simulink model "RoboBoat_SS_July3_v6"  (R2014a)
settings: Solver=FixedStepDiscrete  StartTime=0.0  StopTime=inf  FixedStep=.1  RelTol=1e-3
undefined symbols (not defined in the file): Com1, Com2, Com3, Com4, DiscIntNeverNeededParam, standard
libraries: xpcseriallib x29, visiontextngfix x25, simulink x20, slrtlib x7, speedgoatlib_IO102 x5, speedgoatlib x1
(part 3 of 5)

== system RoboBoat_SS_July3_v6/Main FSM/Obstacle Navigation1/Enter Gate/Gate 2 (White & White) ==
  Sensors : Inport
  RGB image : Inport  Port=2
  Enable : EnablePort  ShowOutputPort=on
  Bus Selector : BusSelector  OutputSignals=Serial In.Buoy Info.Probability,Serial In.Buoy Info.Color ID,Serial In.Buoy Info.Distance,Serial In.Buoy Info.Angle,Serial In.Compass.Heading,Serial In.GPS.latitude,Serial In.GPS.longitude
  Compare To Constant : simulink/Logic and Bit Operations/Compare To Constant  relop=<=  const=2  OutDataTypeStr=boolean
  Compare To Constant1 : simulink/Logic and Bit Operations/Compare To Constant  relop=>=  const=120  OutDataTypeStr=boolean
  Data Type Conversion2 : DataTypeConversion  OutDataTypeStr=double
  Discrete-Time Integrator : DiscreteIntegrator  SampleTime=.1  ICPrevOutput=DiscIntNeverNeededParam  ICPrevScaledInput=DiscIntNeverNeededParam
  Distance : MATLAB Function  TreatAsAtomicUnit=on
  Insert Text : visiontextngfix/Insert Text  inputType=Obsolete  theText='Enter Gate 2'  getTextLocFrom=Specify via dialog  textLoc=[1 1]  getTextColorFrom=Specify via dialog  textColor=[0 0 0]  getTextIntensityFrom=Specify via dialog  textIntensity=0  getTextOpacityFrom=Specify via dialog  textOpacity=1.0  dummyVar2=0  dummyVar3=0  dummyVar4=0  imagePorts=One multidimensional signal  isInputTransposed=off  fontFace=LucidaSansRegular  dummyVar1=0  blockFontSize=12  antiAliased=on
  Logical Operator : Logic  Operator=OR  AllPortsSameDT=off  OutDataTypeStr=boolean
  MATLAB Function : MATLAB Function  TreatAsAtomicUnit=on
  Output Heirarchy : Subsystem
  Outputs : Outport
  wires:
  Output Heirarchy/1(Outputs) -> Outputs/1
  Sensors/1 -> Output Heirarchy/2(Sensors), Bus Selector/1
  Bus Selector/1 -> MATLAB Function/1(Prob)  "<Probability>"
  Bus Selector/2 -> MATLAB Function/2(ColorID)  "<Color ID>"
  Bus Selector/3 -> MATLAB Function/3(Dist)  "<Distance>"
  Bus Selector/4 -> MATLAB Function/4(Ang)  "<Angle>"
  Bus Selector/5 -> MATLAB Function/5(CurrentHeading)  "<Heading>"
  Enable/1 -> Discrete-Time Integrator/1
  Discrete-Time Integrator/1 -> Compare To Constant1/1, MATLAB Function/8(Timer)
  MATLAB Function/1(RPM) -> Output Heirarchy/3(RPM)
  MATLAB Function/2(DesiredHeading) -> Output Heirarchy/4(Desired Heading)
  Bus Selector/6 -> MATLAB Function/6(GPSLat), Distance/2(GPSLat)  "<latitude>"
  Bus Selector/7 -> MATLAB Function/7(GPSLong), Distance/3(GPSLong)  "<longitude>"
  Distance/1(Distance) -> Compare To Constant/1
  RGB image/1 -> Insert Text/1
  Data Type Conversion2/1 -> Output Heirarchy/5(Task Finished)
  Compare To Constant/1 -> Logical Operator/2
  MATLAB Function/3(gateGPS) -> Distance/1(DesiredGPS)
  Compare To Constant1/1 -> Logical Operator/1
  Logical Operator/1 -> Data Type Conversion2/1
  Insert Text/1 -> Output Heirarchy/1(Annotated Image)

== system RoboBoat_SS_July3_v6/Main FSM/Obstacle Navigation1/Enter Gate/Gate 3 (White & Green) ==
  Sensors : Inport
  RGB image : Inport  Port=2
  Enable : EnablePort  ShowOutputPort=on
  Bus Selector : BusSelector  OutputSignals=Serial In.Buoy Info.Probability,Serial In.Buoy Info.Color ID,Serial In.Buoy Info.Distance,Serial In.Buoy Info.Angle,Serial In.Compass.Heading,Serial In.GPS.latitude,Serial In.GPS.longitude
  Compare To Constant : simulink/Logic and Bit Operations/Compare To Constant  relop=<=  const=2  OutDataTypeStr=boolean
  Compare To Constant1 : simulink/Logic and Bit Operations/Compare To Constant  relop=>=  const=120  OutDataTypeStr=boolean
  Data Type Conversion2 : DataTypeConversion  OutDataTypeStr=double
  Discrete-Time Integrator : DiscreteIntegrator  SampleTime=.1  ICPrevOutput=DiscIntNeverNeededParam  ICPrevScaledInput=DiscIntNeverNeededParam
  Distance : MATLAB Function  TreatAsAtomicUnit=on
  Insert Text : visiontextngfix/Insert Text  inputType=Obsolete  theText='Enter Gate 3'  getTextLocFrom=Specify via dialog  textLoc=[1 1]  getTextColorFrom=Specify via dialog  textColor=[0 0 0]  getTextIntensityFrom=Specify via dialog  textIntensity=0  getTextOpacityFrom=Specify via dialog  textOpacity=1.0  dummyVar2=0  dummyVar3=0  dummyVar4=0  imagePorts=One multidimensional signal  isInputTransposed=off  fontFace=LucidaSansRegular  dummyVar1=0  blockFontSize=12  antiAliased=on
  Logical Operator : Logic  Operator=OR  AllPortsSameDT=off  OutDataTypeStr=boolean
  MATLAB Function : MATLAB Function  TreatAsAtomicUnit=on
  Output Heirarchy : Subsystem
  Outputs : Outport
  wires:
  Output Heirarchy/1(Outputs) -> Outputs/1
  Sensors/1 -> Output Heirarchy/2(Sensors), Bus Selector/1
  Bus Selector/1 -> MATLAB Function/1(Prob)  "<Probability>"
  Bus Selector/2 -> MATLAB Function/2(ColorID)  "<Color ID>"
  Bus Selector/3 -> MATLAB Function/3(Dist)  "<Distance>"
  Bus Selector/4 -> MATLAB Function/4(Ang)  "<Angle>"
  Bus Selector/5 -> MATLAB Function/5(CurrentHeading)  "<Heading>"
  Enable/1 -> Discrete-Time Integrator/1
  Discrete-Time Integrator/1 -> Compare To Constant1/1, MATLAB Function/8(Timer)
  MATLAB Function/1(RPM) -> Output Heirarchy/3(RPM)
  MATLAB Function/2(DesiredHeading) -> Output Heirarchy/4(Desired Heading)
  Bus Selector/6 -> MATLAB Function/6(GPSLat), Distance/2(GPSLat)  "<latitude>"
  Bus Selector/7 -> MATLAB Function/7(GPSLong), Distance/3(GPSLong)  "<longitude>"
  Distance/1(Distance) -> Compare To Constant/1
  RGB image/1 -> Insert Text/1
  Data Type Conversion2/1 -> Output Heirarchy/5(Task Finished)
  Compare To Constant/1 -> Logical Operator/2
  MATLAB Function/3(gateGPS) -> Distance/1(DesiredGPS)
  Compare To Constant1/1 -> Logical Operator/1
  Logical Operator/1 -> Data Type Conversion2/1
  Insert Text/1 -> Output Heirarchy/1(Annotated Image)

== system RoboBoat_SS_July3_v6/Main FSM/Obstacle Navigation1/Enter Gate/Output Reassign ==
  Outputs in : Inport
  Bus Assignment : BusAssignment  AssignedSignals=Task Finished
  Bus Selector : BusSelector  OutputSignals=Task Finished
  Constant : Constant  Value=0
  Outputs : Outport
  Finished : Outport  Port=2
  wires:
  Outputs in/1 -> Bus Assignment/1, Bus Selector/1
  Bus Selector/1 -> Finished/1  "<Task Finished>"
  Bus Assignment/1 -> Outputs/1
  Constant/1 -> Bus Assignment/2

== system RoboBoat_SS_July3_v6/Main FSM/Obstacle Navigation1/Exit Gate/Gate 1 (Red & White) ==
  Sensors : Inport
  RGB image : Inport  Port=2
  Enable : EnablePort  ShowOutputPort=on
  Bus Selector : BusSelector  OutputSignals=Serial In.Buoy Info.Probability,Serial In.Buoy Info.Color ID,Serial In.Buoy Info.Distance,Serial In.Buoy Info.Angle,Serial In.Compass.Heading,Serial In.GPS.latitude,Serial In.GPS.longitude
  Compare To Constant : simulink/Logic and Bit Operations/Compare To Constant  relop=<=  const=2  OutDataTypeStr=boolean
  Compare To Constant1 : simulink/Logic and Bit Operations/Compare To Constant  relop=>=  const=120  OutDataTypeStr=boolean
  Data Type Conversion2 : DataTypeConversion  OutDataTypeStr=double
  Discrete-Time Integrator : DiscreteIntegrator  SampleTime=.1  ICPrevOutput=DiscIntNeverNeededParam  ICPrevScaledInput=DiscIntNeverNeededParam
  Distance : MATLAB Function  TreatAsAtomicUnit=on
  Insert Text : visiontextngfix/Insert Text  inputType=Obsolete  theText='Exit Gate 1'  getTextLocFrom=Specify via dialog  textLoc=[1 1]  getTextColorFrom=Specify via dialog  textColor=[0 0 0]  getTextIntensityFrom=Specify via dialog  textIntensity=0  getTextOpacityFrom=Specify via dialog  textOpacity=1.0  dummyVar2=0  dummyVar3=0  dummyVar4=0  imagePorts=One multidimensional signal  isInputTransposed=off  fontFace=LucidaSansRegular  dummyVar1=0  blockFontSize=12  antiAliased=on
  Logical Operator : Logic  Operator=OR  AllPortsSameDT=off  OutDataTypeStr=boolean
  MATLAB Function : MATLAB Function  TreatAsAtomicUnit=on
  Output Heirarchy : Subsystem
  Outputs : Outport
  wires:
  Output Heirarchy/1(Outputs) -> Outputs/1
  Sensors/1 -> Output Heirarchy/2(Sensors), Bus Selector/1
  Bus Selector/1 -> MATLAB Function/1(Prob)  "<Probability>"
  Bus Selector/2 -> MATLAB Function/2(ColorID)  "<Color ID>"
  Bus Selector/3 -> MATLAB Function/3(Dist)  "<Distance>"
  Bus Selector/4 -> MATLAB Function/4(Ang)  "<Angle>"
  Bus Selector/5 -> MATLAB Function/5(CurrentHeading)  "<Heading>"
  Enable/1 -> Discrete-Time Integrator/1
  Discrete-Time Integrator/1 -> Compare To Constant1/1, MATLAB Function/8(Timer)
  MATLAB Function/1(RPM) -> Output Heirarchy/3(RPM)
  MATLAB Function/2(DesiredHeading) -> Output Heirarchy/4(Desired Heading)
  Bus Selector/6 -> MATLAB Function/6(GPSLat), Distance/2(GPSLat)  "<latitude>"
  Bus Selector/7 -> MATLAB Function/7(GPSLong), Distance/3(GPSLong)  "<longitude>"
  Distance/1(Distance) -> Compare To Constant/1
  RGB image/1 -> Insert Text/1
  Insert Text/1 -> Output Heirarchy/1(Annotated Image)
  Data Type Conversion2/1 -> Output Heirarchy/5(Task Finished)
  Compare To Constant/1 -> Logical Operator/2
  MATLAB Function/3(gateGPS) -> Distance/1(DesiredGPS)
  Compare To Constant1/1 -> Logical Operator/1
  Logical Operator/1 -> Data Type Conversion2/1

== system RoboBoat_SS_July3_v6/Main FSM/Obstacle Navigation1/Exit Gate/Gate 2 (White & White) ==
  Sensors : Inport
  RGB image : Inport  Port=2
  Enable : EnablePort  ShowOutputPort=on
  Bus Selector : BusSelector  OutputSignals=Serial In.Buoy Info.Probability,Serial In.Buoy Info.Color ID,Serial In.Buoy Info.Distance,Serial In.Buoy Info.Angle,Serial In.Compass.Heading,Serial In.GPS.latitude,Serial In.GPS.longitude
  Compare To Constant : simulink/Logic and Bit Operations/Compare To Constant  relop=<=  const=2  OutDataTypeStr=boolean
  Compare To Constant1 : simulink/Logic and Bit Operations/Compare To Constant  relop=>=  const=120  OutDataTypeStr=boolean
  Data Type Conversion2 : DataTypeConversion  OutDataTypeStr=double
  Discrete-Time Integrator : DiscreteIntegrator  SampleTime=.1  ICPrevOutput=DiscIntNeverNeededParam  ICPrevScaledInput=DiscIntNeverNeededParam
  Distance : MATLAB Function  TreatAsAtomicUnit=on
  Insert Text : visiontextngfix/Insert Text  inputType=Obsolete  theText='Exit Gate 2'  getTextLocFrom=Specify via dialog  textLoc=[1 1]  getTextColorFrom=Specify via dialog  textColor=[0 0 0]  getTextIntensityFrom=Specify via dialog  textIntensity=0  getTextOpacityFrom=Specify via dialog  textOpacity=1.0  dummyVar2=0  dummyVar3=0  dummyVar4=0  imagePorts=One multidimensional signal  isInputTransposed=off  fontFace=LucidaSansRegular  dummyVar1=0  blockFontSize=12  antiAliased=on
  Logical Operator : Logic  Operator=OR  AllPortsSameDT=off  OutDataTypeStr=boolean
  MATLAB Function : MATLAB Function  TreatAsAtomicUnit=on
  Output Heirarchy : Subsystem
  Outputs : Outport
  wires:
  Output Heirarchy/1(Outputs) -> Outputs/1
  Sensors/1 -> Output Heirarchy/2(Sensors), Bus Selector/1
  Bus Selector/1 -> MATLAB Function/1(Prob)  "<Probability>"
  Bus Selector/2 -> MATLAB Function/2(ColorID)  "<Color ID>"
  Bus Selector/3 -> MATLAB Function/3(Dist)  "<Distance>"
  Bus Selector/4 -> MATLAB Function/4(Ang)  "<Angle>"
  Bus Selector/5 -> MATLAB Function/5(CurrentHeading)  "<Heading>"
  Enable/1 -> Discrete-Time Integrator/1
  Discrete-Time Integrator/1 -> Compare To Constant1/1, MATLAB Function/8(Timer)
  MATLAB Function/1(RPM) -> Output Heirarchy/3(RPM)
  MATLAB Function/2(DesiredHeading) -> Output Heirarchy/4(Desired Heading)
  Bus Selector/6 -> MATLAB Function/6(GPSLat), Distance/2(GPSLat)  "<latitude>"
  Bus Selector/7 -> MATLAB Function/7(GPSLong), Distance/3(GPSLong)  "<longitude>"
  Distance/1(Distance) -> Compare To Constant/1
  RGB image/1 -> Insert Text/1
  Data Type Conversion2/1 -> Output Heirarchy/5(Task Finished)
  Compare To Constant/1 -> Logical Operator/2
  MATLAB Function/3(gateGPS) -> Distance/1(DesiredGPS)
  Compare To Constant1/1 -> Logical Operator/1
  Logical Operator/1 -> Data Type Conversion2/1
  Insert Text/1 -> Output Heirarchy/1(Annotated Image)

== system RoboBoat_SS_July3_v6/Main FSM/Obstacle Navigation1/Exit Gate/Gate 3 (White & Green) ==
  Sensors : Inport
  RGB image : Inport  Port=2
  Enable : EnablePort  ShowOutputPort=on
  Bus Selector : BusSelector  OutputSignals=Serial In.Buoy Info.Probability,Serial In.Buoy Info.Color ID,Serial In.Buoy Info.Distance,Serial In.Buoy Info.Angle,Serial In.Compass.Heading,Serial In.GPS.latitude,Serial In.GPS.longitude
  Compare To Constant : simulink/Logic and Bit Operations/Compare To Constant  relop=<=  const=2  OutDataTypeStr=boolean
  Compare To Constant1 : simulink/Logic and Bit Operations/Compare To Constant  relop=>=  const=120  OutDataTypeStr=boolean
  Data Type Conversion2 : DataTypeConversion  OutDataTypeStr=double
  Discrete-Time Integrator : DiscreteIntegrator  SampleTime=.1  ICPrevOutput=DiscIntNeverNeededParam  ICPrevScaledInput=DiscIntNeverNeededParam
  Distance : MATLAB Function  TreatAsAtomicUnit=on
  Insert Text : visiontextngfix/Insert Text  inputType=Obsolete  theText='Exit Gate 3'  getTextLocFrom=Specify via dialog  textLoc=[1 1]  getTextColorFrom=Specify via dialog  textColor=[0 0 0]  getTextIntensityFrom=Specify via dialog  textIntensity=0  getTextOpacityFrom=Specify via dialog  textOpacity=1.0  dummyVar2=0  dummyVar3=0  dummyVar4=0  imagePorts=One multidimensional signal  isInputTransposed=off  fontFace=LucidaSansRegular  dummyVar1=0  blockFontSize=12  antiAliased=on
  Logical Operator : Logic  Operator=OR  AllPortsSameDT=off  OutDataTypeStr=boolean
  MATLAB Function : MATLAB Function  TreatAsAtomicUnit=on
  Output Heirarchy : Subsystem
  Outputs : Outport
  wires:
  Output Heirarchy/1(Outputs) -> Outputs/1
  Sensors/1 -> Output Heirarchy/2(Sensors), Bus Selector/1
  Bus Selector/1 -> MATLAB Function/1(Prob)  "<Probability>"
  Bus Selector/2 -> MATLAB Function/2(ColorID)  "<Color ID>"
  Bus Selector/3 -> MATLAB Function/3(Dist)  "<Distance>"
  Bus Selector/4 -> MATLAB Function/4(Ang)  "<Angle>"
  Bus Selector/5 -> MATLAB Function/5(CurrentHeading)  "<Heading>"
  Enable/1 -> Discrete-Time Integrator/1
  Discrete-Time Integrator/1 -> Compare To Constant1/1, MATLAB Function/8(Timer)
  MATLAB Function/1(RPM) -> Output Heirarchy/3(RPM)
  MATLAB Function/2(DesiredHeading) -> Output Heirarchy/4(Desired Heading)
  Bus Selector/6 -> MATLAB Function/6(GPSLat), Distance/2(GPSLat)  "<latitude>"
  Bus Selector/7 -> MATLAB Function/7(GPSLong), Distance/3(GPSLong)  "<longitude>"
  Distance/1(Distance) -> Compare To Constant/1
  RGB image/1 -> Insert Text/1
  Data Type Conversion2/1 -> Output Heirarchy/5(Task Finished)
  Compare To Constant/1 -> Logical Operator/2
  MATLAB Function/3(gateGPS) -> Distance/1(DesiredGPS)
  Compare To Constant1/1 -> Logical Operator/1
  Logical Operator/1 -> Data Type Conversion2/1
  Insert Text/1 -> Output Heirarchy/1(Annotated Image)

== system RoboBoat_SS_July3_v6/Main FSM/Obstacle Navigation1/GPS: Center/Approach ==
  Sensors : Inport
  RGB image : Inport  Port=2
  Enable : EnablePort
  Annotate Task : visiontextngfix/Insert Text  inputType=Obsolete  theText='GPS - Center: Approach - Distance: %f'  getTextLocFrom=Specify via dialog  textLoc=[10 70]  getTextColorFrom=Specify via dialog  textColor=[255 0 0]  getTextIntensityFrom=Specify via dialog  textIntensity=0  getTextOpacityFrom=Specify via dialog  textOpacity=1.0  dummyVar2=0  dummyVar3=0  dummyVar4=0  imagePorts=One multidimensional signal  isInputTransposed=off  fontFace=LucidaSansRegular  dummyVar1=0  blockFontSize=12  antiAliased=on
  Annotate Task2 : visiontextngfix/Insert Text  inputType=Obsolete  theText='Obst Nav Start'  getTextLocFrom=Specify via dialog  textLoc=[1 1]  getTextColorFrom=Specify via dialog  textColor=[0 0 0]  getTextIntensityFrom=Specify via dialog  textIntensity=0  getTextOpacityFrom=Specify via dialog  textOpacity=1.0  dummyVar2=0  dummyVar3=0  dummyVar4=0  imagePorts=One multidimensional signal  isInputTransposed=off  fontFace=LucidaSansRegular  dummyVar1=0  blockFontSize=12  antiAliased=on
  Bus Selector : BusSelector  OutputSignals=Serial In.GPS.latitude,Serial In.GPS.longitude
  Compare To Constant : simulink/Logic and Bit Operations/Compare To Constant  relop=<=  const=5  OutDataTypeStr=boolean
  Data Store Read : DataStoreRead  DataStoreName=obstNavStartGPS  SampleTime=0.1
  Data Type Conversion : DataTypeConversion  OutDataTypeStr=double
  Desired Heading and Distance : MATLAB Function  TreatAsAtomicUnit=on
  MATLAB Function : MATLAB Function  Commented=on  TreatAsAtomicUnit=on
  Output Heirarchy : Subsystem
  "Scope " : slrtlib/Displays and Logging/Scope   Commented=on  scopeno=1  scopetype=File  autostart=on  viewmode=Graphical redraw  formatstr='%15.6f'  grid=on  ylimits=[0,0]  nosamples=1200  noprepostsamples=0  interleave=1  triggermode=FreeRun  triggersignal=1  trigsignalfromport=off  triggerlevel=1  triggerslope=Either  triggerscope=1  triggersample=0  filename=ApprLog.dat  mode=Lazy  writesize=512  autorestart=off  dynamicfilemode=off  maxwritefilesize=512*1024^2
  Outputs : Outport
  wires:
  Sensors/1 -> Output Heirarchy/4(Sensors), Bus Selector/1  "Sensors"
  Data Store Read/1 -> Desired Heading and Distance/1(DesiredGPS)
  Bus Selector/1 -> Desired Heading and Distance/2(GPSLat)  "<latitude>"
  Bus Selector/2 -> Desired Heading and Distance/3(GPSLong)  "<longitude>"
  Desired Heading and Distance/2(DesiredHeading) -> Output Heirarchy/2(Desired Heading)
  Annotate Task/1 -> Output Heirarchy/3(Annotated Image)
  RGB image/1 -> Annotate Task2/1
  Output Heirarchy/1(Outputs) -> Outputs/1
  Annotate Task2/1 -> Annotate Task/1
  MATLAB Function/1(out) -> "Scope "/1
  Desired Heading and Distance/1(Distance) -> Compare To Constant/1, Annotate Task/2
  Data Type Conversion/1 -> Output Heirarchy/1(Finished)  "Task Finished"
  Compare To Constant/1 -> Data Type Conversion/1

== system RoboBoat_SS_July3_v6/Main FSM/Obstacle Navigation1/GPS: Center/Orient ==
  Sensors : Inport
  RGB image : Inport  Port=2
  Enable : EnablePort
  Annotate Task : visiontextngfix/Insert Text  inputType=Obsolete  theText='GPS - Center: Orient %f'  getTextLocFrom=Specify via dialog  textLoc=[10 70]  getTextColorFrom=Specify via dialog  textColor=[255 0 0]  getTextIntensityFrom=Specify via dialog  textIntensity=0  getTextOpacityFrom=Specify via dialog  textOpacity=1.0  dummyVar2=0  dummyVar3=0  dummyVar4=0  imagePorts=One multidimensional signal  isInputTransposed=off  fontFace=LucidaSansRegular  dummyVar1=0  blockFontSize=12  antiAliased=on
  Annotate Task1 : visiontextngfix/Insert Text  inputType=Obsolete  theText='Current Heading %f'  getTextLocFrom=Specify via dialog  textLoc=[10 40]  getTextColorFrom=Specify via dialog  textColor=[255 0 0]  getTextIntensityFrom=Specify via dialog  textIntensity=0  getTextOpacityFrom=Specify via dialog  textOpacity=1.0  dummyVar2=0  dummyVar3=0  dummyVar4=0  imagePorts=One multidimensional signal  isInputTransposed=off  fontFace=LucidaSansRegular  dummyVar1=0  blockFontSize=12  antiAliased=on
  Annotate Task2 : visiontextngfix/Insert Text  inputType=Obsolete  theText='Obst Nav Start'  getTextLocFrom=Specify via dialog  textLoc=[1 1]  getTextColorFrom=Specify via dialog  textColor=[0 0 0]  getTextIntensityFrom=Specify via dialog  textIntensity=0  getTextOpacityFrom=Specify via dialog  textOpacity=1.0  dummyVar2=0  dummyVar3=0  dummyVar4=0  imagePorts=One multidimensional signal  isInputTransposed=off  fontFace=LucidaSansRegular  dummyVar1=0  blockFontSize=12  antiAliased=on
  Bus Selector : BusSelector  OutputSignals=Serial In.GPS.latitude,Serial In.GPS.longitude,Serial In.Compass.Heading
  Data Store Read : DataStoreRead  DataStoreName=obstNavStartGPS  SampleTime=0.1
  Desired Heading : MATLAB Function  TreatAsAtomicUnit=on
  Output Heirarchy1 : Subsystem
  Within Range : MATLAB Function  TreatAsAtomicUnit=on
  Outputs : Outport
  Finished : Outport  Port=2
  wires:
  Sensors/1 -> Output Heirarchy1/3(Sensors), Bus Selector/1  "Sensors"
  Data Store Read/1 -> Desired Heading/1(DesiredGPS)
  Bus Selector/1 -> Desired Heading/2(GPSLat)  "<latitude>"
  Bus Selector/2 -> Desired Heading/3(GPSLong)  "<longitude>"
  Desired Heading/1(DesiredHeading) -> Output Heirarchy1/2(Desired Heading), Annotate Task/2, Within Range/1(DesiredHeading)
  Bus Selector/3 -> Annotate Task1/2, Within Range/2(Compass)  "<Heading>"
  Within Range/1(Finished) -> Finished/1
  RGB image/1 -> Annotate Task2/1
  Output Heirarchy1/1(Outputs) -> Outputs/1
  Annotate Task/1 -> Annotate Task1/1
  Annotate Task1/1 -> Output Heirarchy1/1(Annotated Image)
  Annotate Task2/1 -> Annotate Task/1

== system RoboBoat_SS_July3_v6/Main FSM/Obstacle Navigation1/GPS: Center/Output Reassign ==
  Outputs in : Inport
  Bus Assignment : BusAssignment  AssignedSignals=Task Finished
  Bus Selector : BusSelector  OutputSignals=Task Finished
  Constant : Constant  Value=0
  Outputs : Outport
  Finished : Outport  Port=2
  wires:
  Outputs in/1 -> Bus Assignment/1, Bus Selector/1
  Bus Selector/1 -> Finished/1  "<Task Finished>"
  Bus Assignment/1 -> Outputs/1
  Constant/1 -> Bus Assignment/2

== matlab function RoboBoat_SS_July3_v6/Main FSM/Obstacle Navigation1/Exit Gate/Gate 3 (White & Green)/Distance ==
  data: Distance output; DesiredGPS input; GPSLat input; GPSLong input
function Distance  = DistCalc(DesiredGPS, GPSLat, GPSLong)

%Written by Anderson Lebbad on July 22, 2013
%Last Edited:

%Orients the boat towards a target GPS point before approaching it.
%This is done to keep the approach angle minimal, so the approach
%algorithm does not circle the target and never reach it.

%Parse input GPS and convert angles to radians
CurLat = (floor(GPSLat/100)+mod(GPSLat,100)/60)*pi/180;
CurLong = (floor(GPSLong/100)+mod(GPSLong,100)/60)*pi/180;
DesLat = (floor(DesiredGPS(1)/100)+mod(DesiredGPS(1),100)/60)*pi/180;
DesLong = (floor(DesiredGPS(2)/100)+mod(DesiredGPS(2),100)/60)*pi/180;
%Difference between lats and longs
DiffLat = DesLat - CurLat;
MidLat = cos((CurLat + DesLat)/2);
DiffLong = DesLong - CurLong;
%Radius of the earth in meters
R = 6378137;

%Calculate distance using the great-circle distance formula
%Formula documented here:
%   http://www.movable-type.co.uk/scripts/latlong.html
% a = sin(DiffLat/2)^2+sin(DiffLong/2)^2*cos(CurLat)*cos(DesLat);
% c = 2*atan2(sqrt(a), sqrt(1-a));
% Distance = R*c;

%Calculating distance using Pythagora's
a = DiffLong*MidLat;
b = DiffLat;
Distance = R*sqrt(a^2+b^2);

== matlab function RoboBoat_SS_July3_v6/Main FSM/Obstacle Navigation1/Exit Gate/MATLAB Function ==
  data: gateID input; outputSelector output; gate1En output; gate2En output; gate3En output
function [outputSelector,gate1En,gate2En,gate3En] = gateSelector(gateID)
% Determines which colors to filter for based on the gateID as received
% from the judges

gate1En = 0;
gate2En = 0;
gate3En = 0;

if gateID == 1
    gate1En = 1;
    outputSelector = 1;
elseif gateID == 2
    gate2En = 1;
    outputSelector = 2;
else
    gate3En = 1;
    outputSelector = 3;
end

== matlab function RoboBoat_SS_July3_v6/Sinks/MATLAB Function1 ==
  data: PortPow input; PortV output; StbdPow input; StbdV output
function [PortV, StbdV] = toVoltage(PortPow,StbdPow)
%Written By Anderson Lebbad on June 19, 2015
%Last Edited by:
%
%This function converts a desired value (0-100%, positive or negative) for
%each thruster to drive voltages.

%Signal is biased by 2.5 as it is voltage neutral, 5v control signal
PortV = -PortPow/100*2.5+2.5;
StbdV = StbdPow/100*2.5+2.5;

end

== matlab function RoboBoat_SS_July3_v6/Main FSM/Start Speed/Gate Find and Through/Find/MATLAB Function1 ==
  data: Dist input; Angles input; X input; Y input; Heading input; found output; Goal output; Color input; idx input
function [found, Goal] = SpeedGate(Dist,Angles,X,Y,Heading,Color,idx)
%Written by Anderson Lebbad on May 29, 2015
%Last Edited by: Anderson Lebbad on July 3, 2015 - green is more likely to
%be seen, so dodge to the left rather than right.

%This function sends theboat forward until a landmark is found, then it
%navigates towards the right of it.

persistent goalX goalY Found %initialHeading change
if isempty(goalX)
    goalX = X;
    goalY = Y;
    Found = 0;
    %     initialHeading = Heading;
    %     change = 10;
end

% DesiredHeading = Heading;
DistM = Dist./100;
dodgeWidth = 3;

if Found == 0
    if idx(2) ~= 0
        %Check colors of objects
        buoy1Green = (Color(1) > 43) && (Color(1) < 128);
        buoy2Green = (Color(2) > 43) && (Color(2) < 128);
        if buoy1Green
            if ~buoy2Green
                %If two objects are found of differing color, set goal between the two
                w = (DistM(9)*sin(Angles(9)*pi/180) + DistM(10)*sin(Angles(10)*pi/180)) / 2;
                h = (DistM(9)*cos(Angles(9)*pi/180) + DistM(10)*sin(Angles(10)*pi/180)) / 2;
            else
                %dodge to the left of green buoy
                w = DistM(9)*sin(Angles(9)*pi/180) - dodgeWidth;
                h = DistM(9)*cos(Angles(9)*pi/180);
            end
        else
            if buoy2Green
                %If two objects are found of differing color, set goal between the two
                w = (DistM(9)*sin(Angles(9)*pi/180) + DistM(10)*sin(Angles(10)*pi/180)) / 2;
                h = (DistM(9)*cos(Angles(9)*pi/180) + DistM(10)*sin(Angles(10)*pi/180)) / 2;
            else
                %dodge to the right of red buoy
                w = DistM(9)*sin(Angles(9)*pi/180) + dodgeWidth;
                h = DistM(9)*cos(Angles(9)*pi/180);
            end
        end
        goalX = X + h*cos(Heading*pi/180) - w*sin(Heading*pi/180);
        goalY = Y + h*sin(Heading*pi/180) + w*cos(Heading*pi/180);
        Found = 1;
    elseif idx(1) ~= 0
        %if color value is less than 110, buoy is identified as green
        if (Color(1) > 43) && (Color(1) < 128)
            %dodge to the left of green buoy
            w = DistM(9)*sin(Angles(9)*pi/180) - dodgeWidth;
        else
            %dodge to the right of red buoy
            w = DistM(9)*sin(Angles(9)*pi/180) + dodgeWidth;
        end
        h = DistM(9)*cos(Angles(9)*pi/180);
        goalX = X + h*cos(Heading*pi/180) - w*sin(Heading*pi/180);
        goalY = Y + h*sin(Heading*pi/180) + w*cos(Heading*pi/180);
        Found = 1;
    else
        %If no objects are found, search. Scan 30 degrees to left and right
        %of initial heading.
        %         DesiredHeading = Heading + change;
        %         if abs(DesiredHeading - initialHeading) > 30
        %             change = -change;
        %             DesiredHeading = Heading + change;
        %         end
    end
end

Goal = [goalX, goalY];
found = Found;

end

== matlab function RoboBoat_SS_July3_v6/Main FSM/Obstacle Navigation1/Enter Gate/Gate 1 (Red & White)/MATLAB Function ==
  data: Prob input; RPM output; ColorID input; Dist input; Ang input; CurrentHeading input; GPSLat input; GPSLong input; Timer input; DesiredHeading output; gateGPS output
function [RPM,DesiredHeading,gateGPS] = navigation(Prob,ColorID,Dist,Ang,CurrentHeading,GPSLat,GPSLong,Timer)

% Function performs one buoy navigation through the start speed gates. If
% no buoys are found by the LIDAR/Vision assembly then an incremented
% turning algorithm is executed to turn by 10 degrees per increment up to 
% 90 degrees either way of the inital heading

% Written by Edward Zhu

persistent LockHeading TimeLastFound Counter Turn TurnInc gateLat gateLong

if isempty(LockHeading) && isempty(TimeLastFound) && isempty(Counter) && isempty(Turn) && isempty(TurnInc)
    LockHeading = CurrentHeading;
    TimeLastFound = 0;
    Counter = 0;
    TurnInc = 30;
    Turn = TurnInc;
    gateLat = 0;
    gateLong = 0;
end

Distance = Dist/100;

BoatWidth = 0.75;
Buffer = atan(2*BoatWidth/Distance);

RedOffset = Ang + Buffer;
WhiteOffset = Ang - Buffer;

R = 6378137;

CurLat = (floor(GPSLat/100)+mod(GPSLat,100)/60)*pi/180;
CurLong = (ceil(GPSLong/100)-mod(-GPSLong,100)/60)*pi/180;

gateHeading = (mod(CurrentHeading + Ang, 360))*pi/180;

if ColorID == 1 && Prob > 0.9
    if Ang < 0
        DesiredHeading = mod(CurrentHeading - RedOffset, 360);
    else
        DesiredHeading = mod(CurrentHeading + RedOffset, 360);
    end
    RPM = 4000;
    GateFound = 1;
    TimeLastFound = Timer;
    gateLat =  asin(sin(CurLat)*cos(Distance/R) + cos(CurLat)*sin(Distance/R)*cos(gateHeading))*180/pi;
    gateLong = (CurLong + atan2(sin(gateHeading)*sin(Distance/R)*cos(CurLat),cos(Distance/R)-sin(CurLat)*sin(gateLat)))*180/pi;
elseif ColorID == 2 && Prob > 0.9
    DesiredHeading = mod(LockHeading - Turn, 360);
    RPM = 0;
    GateFound = 1;
    TimeLastFound = Timer;
%     DesiredHeading = mod(CurrentHeading - WhiteOffset, 360);
%     RPM = 4000;
%     GateFound = 1;
%     TimeLastFound = Timer;
%     gateLat =  asin(sin(CurLat)*cos(Distance/R) + cos(CurLat)*sin(Distance/R)*cos(gateHeading))*180/pi;
%     gateLong = (CurLong + atan2(sin(gateHeading)*sin(Distance/R)*cos(CurLat),cos(Distance/R)-sin(CurLat)*sin(gateLat)))*180/pi;
else
    DesiredHeading = CurrentHeading;
    RPM = 0;
    GateFound = 0;
end

gateGPS = [gateLat gateLong];
TimeNoBuoys = Timer - TimeLastFound;

if GateFound == 0 && TimeNoBuoys > 15
    RPM = 0;
    DesiredHeading = mod(LockHeading - Turn, 360);
    HeadingDiff = DesiredHeading - CurrentHeading;
    gateGPS = [gateLat gateLong];
    
    if HeadingDiff > 180
        HeadingDiff = HeadingDiff - 360;
    elseif HeadingDiff < -180
        HeadingDiff = HeadingDiff + 360;
    end
    
    if HeadingDiff < 3
        Counter = Counter + 1;
    else
        Counter = 0;
    end
    
    if Counter >= 15
        Turn = Turn + TurnInc;
        Counter = 0;
        if abs(Turn) > 90
            TurnInc = -TurnInc;
        end
    end
end

== matlab function RoboBoat_SS_July3_v6/Main FSM/Obstacle Navigation1/Enter Gate/MATLAB Function ==
  data: gateID input; outputSelector output; gate1En output; gate2En output; gate3En output
function [outputSelector,gate1En,gate2En,gate3En] = gateSelector(gateID)
% Determines which colors to filter for based on the gateID as received
% from the judges

gate1En = 0;
gate2En = 0;
gate3En = 0;

if gateID == 1
    gate1En = 1;
    outputSelector = 1;
elseif gateID == 2
    gate2En = 1;
    outputSelector = 2;
else
    gate3En = 1;
    outputSelector = 3;
end

== matlab function RoboBoat_SS_July3_v6/Main FSM/Start Speed/Gate Find and Through/Point/MATLAB Function1 ==
  data: holdHeading input; yaw input; finished output
function finished  = aimed(holdHeading,yaw)
%Written by Anderson Lebbad on May 29, 2015
%Last Edited by: Anderson Lebbad on July 3, 2015 for count

%This function sends theboat forward until a landmark is found, then it
%navigates towards the right of it.

persistent count
if isempty(count)
    count = 0;
end

%initialize output
finished = 0;

%heading difference
headingDiff = holdHeading - yaw;
headingDiff = atan2(sin(headingDiff*pi/180),cos(headingDiff*pi/180))*180/pi;

if abs(headingDiff) < 5
    count = count + 1;
else
    count = 0;
end

%Make sure held heading is stable
if count > 10
    finished = 1;
end

end

== matlab function RoboBoat_SS_July3_v6/Main FSM/Obstacle Navigation1/Obstacle Navigation/GPS: Bee Line/Orient/Within Range ==
  data: DesiredHeading input; Finished output; Compass input
function Finished = OrientLocked(DesiredHeading, Compass)

%Written by Anderson Lebbad on July 22, 2013
%Last Edited:

%This function checks to see if the target heading has been reached and 
%sends a finished signal when it has.

HeadingDiff = DesiredHeading - Compass;

%Sets the range for the difference angle to be -180 to +180
if HeadingDiff > 180
    HeadingDiff = HeadingDiff - 360;
elseif HeadingDiff < -180
    HeadingDiff = HeadingDiff + 360;
end

%If the Heading is within 3 degrees, the angle is close enough to send a
%finished signal
if abs(HeadingDiff) < 3
    Finished = 1;
else
    Finished = 0;
end

== matlab function RoboBoat_SS_July3_v6/Main FSM/Obstacle Navigation1/GPS: Center/Approach/MATLAB Function ==
  data: GPSLat input; out output; GPSLong input; IMULat input; IMULong input
function out = dataFormat(GPSLat, GPSLong, IMULat, IMULong)
%#codegen
out = [GPSLat GPSLong IMULat IMULong];

== matlab function RoboBoat_SS_July3_v6/Main FSM/Obstacle Navigation1/GPS: Center/GPS Enabler ==
  data: Finished input; GPSMode output; OrientEnable output; ApproachEnable output
function [GPSMode, OrientEnable, ApproachEnable] =...
    GPSEnable(Finished)

%Written by Anderson Lebbad on July 22, 2013
%Last Edited: July 27, 2013
%   Removed Termination Block

%This function enables GPS tasks. First the boat orients towards the
%target, then it approaches it.


%Parse Finished signal
OrientFinished = Finished(1);


%Initialize Enablers
OrientEnable = 0;
ApproachEnable = 0;


%Switches the enable signal based on which task is flagged as done.
if OrientFinished == 0
    OrientEnable = 1;
    GPSMode = 1;
else
    ApproachEnable = 1;
    GPSMode = 2;
end

== matlab function RoboBoat_SS_July3_v6/Main FSM/Obstacle Navigation1/GPS: Center/Orient/Within Range ==
  data: DesiredHeading input; Finished output; Compass input
function Finished = OrientLocked(DesiredHeading, Compass)

%Written by Anderson Lebbad on July 22, 2013
%Last Edited:

%This function checks to see if the target heading has been reached and 
%sends a finished signal when it has.

HeadingDiff = DesiredHeading - Compass;

%Sets the range for the difference angle to be -180 to +180
if HeadingDiff > 180
    HeadingDiff = HeadingDiff - 360;
elseif HeadingDiff < -180
    HeadingDiff = HeadingDiff + 360;
end

%If the Heading is within 3 degrees, the angle is close enough to send a
%finished signal
if abs(HeadingDiff) < 3
    Finished = 1;
else
    Finished = 0;
end

== matlab function RoboBoat_SS_July3_v6/Main FSM/Obstacle Navigation1/Obstacle Navigation/Dodge/Nav Logic ==
  data: CurrentHeading input; Dist input; Ang input; ObstDist output; RPM output; DesiredHeading output; Timer input; Timeout input; DodgeIncomplete output
 function [ObstDist, RPM, DesiredHeading, DodgeIncomplete] = NavLogic(CurrentHeading,...
    Dist, Ang, Timer, Timeout)

%Written by Anderson Lebbad on August 20, 2013
%Last Edited by:

%Determines the signals for driving through the buoy channel based on the
%bounding box and centroid signals from both the red and green detection
%blocks.

persistent TimeLastFound heldHeading

ObstDist = Dist / 100;

if isempty(TimeLastFound) && isempty(heldHeading)
    TimeLastFound = 0;
    heldHeading = CurrentHeading;
end

if ObstDist > 0 && ObstDist <= 2
    %Buffer for single buoy offset is the angle to twice the boat's width off of the
    %center of the buoy
    BoatWidth = .75;
    Buffer = atan(2 * BoatWidth / ObstDist) * 180 / pi;
    
    if Ang < 0
        ObstOffset = Ang + Buffer;
    else
        ObstOffset = Ang - Buffer;
    end
    
    DesiredHeading = mod(CurrentHeading + ObstOffset, 360);
    RPM = 2800;
    
    TimeLastFound = Timer;
    heldHeading = CurrentHeading;
    
    DodgeIncomplete = 1;
    
else
    DesiredHeading = heldHeading;
    RPM = 2800;
    
    if Timer-TimeLastFound < Timeout
        DodgeIncomplete = 1;
    else
        DodgeIncomplete = 0;
    end

end

== matlab function RoboBoat_SS_July3_v6/Sensors/1020 Comms/Data Update1 ==
  data: Valid input; ControlMode input; V output; C output; L output; A output; Data input; D1 output; D2 output; D3 output; D4 output; D5 output; D6 output; D7 output; D8 output; D9 output; D10 output; D11 output; D12 output; D13 output; D14 output; D15 output; D16 output; D17 output; D18 output; D19 output; D20 output; D21 output; D22 output; D23 output; D24 output; Activate input
function [V,C,L,A,D1,D2,D3,D4,D5,D6,D7,D8,D9,D10,D11,D12,D13,D14,D15,D16,D17,...
    D18,D19,D20,D21,D22,D23,D24] = dataSplit(Valid,ControlMode,Data,Activate)
%Written by Anderson Lebbad on August 10, 2014
%Last Edited by: Anderson Lebbad on September 11, 2014

%This function splits the data vector into the twelve channels it is
%composed of for communication

persistent HoldData

A = Activate;

if isempty(HoldData)
    HoldData = zeros(26,1);
end

L = 8;

if Valid == 1
    HoldData(1) = Valid;
    HoldData(2) = ControlMode;
    HoldData(3) = Data(1);
    HoldData(4) = Data(2);
    HoldData(5) = Data(3);
    HoldData(6) = Data(4);
    HoldData(7) = Data(5);
    HoldData(8) = Data(6);
    HoldData(9) = Data(7);
    HoldData(10) = Data(8);
    HoldData(11) = Data(9);
    HoldData(12) = Data(10);
    HoldData(13) = Data(11);
    HoldData(14) = Data(12);
    HoldData(15) = Data(13);
    HoldData(16) = Data(14);
    HoldData(17) = Data(15);
    HoldData(18) = Data(16);
    HoldData(19) = Data(17);
    HoldData(20) = Data(18);
    HoldData(21) = Data(19);
    HoldData(22) = Data(20);
    HoldData(23) = Data(21);
    HoldData(24) = Data(22);
    HoldData(25) = Data(23);
    HoldData(26) = Data(24);
end

V = HoldData(1);
C = HoldData(2);
D1 = HoldData(3);
D2 = HoldData(4);
D3 = HoldData(5);
D4 = HoldData(6);
D5 = HoldData(7);
D6 = HoldData(8);
D7 = HoldData(9);
D8 = HoldData(10);
D9 = HoldData(11);
D10 = HoldData(12);
D11 = HoldData(13);
D12 = HoldData(14);
D13 = HoldData(15);
D14 = HoldData(16);
D15 = HoldData(17);
D16 = HoldData(18);
D17 = HoldData(19);
D18 = HoldData(20);
D19 = HoldData(21);
D20 = HoldData(22);
D21 = HoldData(23);
D22 = HoldData(24);
D23 = HoldData(25);
D24 = HoldData(26);

end

== matlab function RoboBoat_SS_July3_v6/Sensors/1020 Comms/MATLAB Function2 ==
  data: Time input; asciiLIT output; Sequence input
% This function creates the light tower message to be sent from 
% Speedgoat in ascii code
% Written by: Edward Zhu
% Date: 9/17/14

function asciiLIT = asciiLITEncoder(Time, Sequence)

% Initialize output message vector as the serial output block expects 128
% character message
asciiLIT = uint8(zeros(1,128));

% Convert static strings to ascii code
asciiMsgID = uint8('$RXLIT,');
asciiComma = uint8(',');
asciiTeamID = uint8('FAUVU,');
asciiMsgEnd = uint8('*');
asciiMsgCRLF = [13 10];

% Convert UTC Time input (hhmmss) into ascii code
asciiTime = uint8(zeros(1,7));
asciiTime(7) = asciiComma;

for timeChar = 1:6
    asciiTime(timeChar) = floor(mod(Time,10^(7-timeChar))/...
        10^(6-timeChar)) + 48;
end

% Convert the light sequece into ascii code (1 = R, 2 = B, 3 = G)
asciiSeq = uint8(zeros(1,4)+32);
asciiSeq(4) = asciiMsgEnd;

if Sequence(1) > 0 && Sequence(2) > 0 && Sequence(3) > 0
    for seqChar = 1:3
        if Sequence(seqChar) == 1
            Sequence(seqChar) = uint8('R');
        elseif Sequence(seqChar) == 2
            Sequence(seqChar) = uint8('B');
        elseif Sequence(seqChar) == 3
            Sequence(seqChar) = uint8('G');
        end
    end
    asciiSeq(1:3) = Sequence;
end

% Concat individual ascii arrays into one array
asciiPreChkSum = cat(2,asciiMsgID,asciiTime,asciiTeamID,asciiSeq);

% Calculate the checksum of the message from the '$' to the '*' and convert
% to hex
chkSum = uint8(0);

for chksumChar = 1:(length(asciiPreChkSum)-2)
    chkSum = bitxor(chkSum,asciiPreChkSum(chksumChar+1));
end

% Convert the checksum to ascii
chkSum = dec2hex(chkSum);
asciiChkSum = uint8(zeros(1,length(chkSum))+32);
for i = 1:length(chkSum)
    asciiChkSum(i) = uint8(chkSum(i));
end

% Concat the checksum and the '/r/n' to the end of the message
asciiPostChkSum = cat(2,asciiPreChkSum,asciiChkSum,asciiMsgCRLF);

% Output the final message
asciiLIT(1:length(asciiPostChkSum)) = asciiPostChkSum;

== matlab function RoboBoat_SS_July3_v6/Main FSM/Obstacle Navigation2/MATLAB Function ==
  data: requestNumOut output; CP input; requestNumIn input; Finished output
function [requestNumOut, Finished] = requestSender(CP, requestNumIn)

persistent counter
if isempty(counter)
    counter = 0;
end

if CP < 1
    requestNumOut = requestNumIn;
    Finished = 0;
else
    counter = counter + 1;
    if counter >= 50
        requestNumOut = 0;
        Finished = 1;
    else
        requestNumOut = requestNumIn;
        Finished = 0;
    end
end

== matlab function RoboBoat_SS_July3_v6/Main FSM/Shotgun Speedgate/MATLAB Function ==
  data: Heading input; LockedHeading output
function LockedHeading = HeadingLock(Heading)

persistent lock

if isempty(lock)
    lock = Heading;
end

LockedHeading = lock;

== matlab function RoboBoat_SS_July3_v6/Main FSM/Shotgun Speedgate/MATLAB Function1 ==
  data: desiredHeading input; out output; Heading input
function out = dataOrganizer(desiredHeading, Heading)
%#codegen

out = [desiredHeading Heading];

== system RoboBoat_SS_July3_v6/Main FSM/Obstacle Navigation1/Obstacle Navigation/Dodge ==
  Sensors : Inport
  RGB image : Inport  Port=2
  Enable : EnablePort  ShowOutputPort=on
  Bus Selector1 : BusSelector  OutputSignals=Serial In.Compass.Heading,Serial In.Buoy Info.Distance,Serial In.Buoy Info.Angle
  Constant : Constant  Value=0
  Constant1 : Constant  Value=2
  Data Store Write : DataStoreWrite  DataStoreName=dodgeStart
  Discrete-Time Integrator : DiscreteIntegrator  SampleTime=0.1  ICPrevOutput=DiscIntNeverNeededParam  ICPrevScaledInput=DiscIntNeverNeededParam
  Insert Text : visiontextngfix/Insert Text  inputType=Obsolete  theText='Dodge'  getTextLocFrom=Specify via dialog  textLoc=[1 1]  getTextColorFrom=Specify via dialog  textColor=[0 0 0]  getTextIntensityFrom=Specify via dialog  textIntensity=0  getTextOpacityFrom=Specify via dialog  textOpacity=1.0  dummyVar2=0  dummyVar3=0  dummyVar4=0  imagePorts=One multidimensional signal  isInputTransposed=off  fontFace=LucidaSansRegular  dummyVar1=0  blockFontSize=12  antiAliased=on
  Insert Text1 : visiontextngfix/Insert Text  inputType=Obsolete  theText='Obstacle Distance: %f'  getTextLocFrom=Specify via dialog  textLoc=[10 70]  getTextColorFrom=Specify via dialog  textColor=[255 0 0]  getTextIntensityFrom=Specify via dialog  textIntensity=0  getTextOpacityFrom=Specify via dialog  textOpacity=1.0  dummyVar2=0  dummyVar3=0  dummyVar4=0  imagePorts=One multidimensional signal  isInputTransposed=off  fontFace=LucidaSansRegular  dummyVar1=0  blockFontSize=12  antiAliased=on
  Nav Logic : MATLAB Function  TreatAsAtomicUnit=on
  Output Heirarchy : Subsystem
  Unit Delay1 : UnitDelay  InitialCondition=1  SampleTime=-1
  Outputs : Outport
  Dodge Incomplete : Outport  Port=2
  wires:
  RGB image/1 -> Insert Text/1
  Sensors/1 -> Output Heirarchy/2(Sensors), Bus Selector1/1
  Bus Selector1/1 -> Nav Logic/1(CurrentHeading)  "<Heading>"
  Enable/1 -> Discrete-Time Integrator/1
  Discrete-Time Integrator/1 -> Nav Logic/4(Timer)
  Constant1/1 -> Nav Logic/5(Timeout)
  Nav Logic/4(DodgeIncomplete) -> Dodge Incomplete/1
  Insert Text/1 -> Insert Text1/1
  Nav Logic/1(ObstDist) -> Insert Text1/2
  Nav Logic/2(RPM) -> Output Heirarchy/3(RPM)
  Nav Logic/3(DesiredHeading) -> Output Heirarchy/4(Desired Heading)
  Output Heirarchy/1(Outputs) -> Outputs/1
  Constant/1 -> Unit Delay1/1
  Unit Delay1/1 -> Data Store Write/1
  Insert Text1/1 -> Output Heirarchy/1(Annotated Image)
  Bus Selector1/2 -> Nav Logic/2(Dist)  "<Distance>"
  Bus Selector1/3 -> Nav Logic/3(Ang)  "<Angle>"

== system RoboBoat_SS_July3_v6/Main FSM/Obstacle Navigation1/Obstacle Navigation/GPS: Bee Line ==
  Sensors : Inport
  RGB image : Inport  Port=2
  Enable : EnablePort
  Approach : Subsystem  TreatAsAtomicUnit=on
  Data Store Write : DataStoreWrite  DataStoreName=dodgeStart
  GPS Enabler : MATLAB Function  TreatAsAtomicUnit=on
  GPS Selector : MultiPortSwitch  Inputs=2
  Orient : Subsystem  TreatAsAtomicUnit=on
  Unit Delay : UnitDelay  SampleTime=-1
  Unit Delay1 : UnitDelay  SampleTime=-1
  Outputs : Outport
  wires:
  Sensors/1 -> Orient/1(Sensors), Approach/1(Sensors)
  GPS Enabler/2(OrientEnable) -> Orient/Enable
  GPS Enabler/3(ApproachEnable) -> Approach/Enable
  Orient/2(Finished) -> Unit Delay/1
  Orient/1(Outputs) -> GPS Selector/2
  Approach/1(Outputs) -> GPS Selector/3
  GPS Enabler/1(GPSMode) -> GPS Selector/1
  Unit Delay/1 -> GPS Enabler/1(Finished)
  RGB image/1 -> Orient/2(RGB image), Approach/2(RGB image)
  Approach/2(Dodge Start) -> Unit Delay1/1
  Unit Delay1/1 -> Data Store Write/1
  GPS Selector/1 -> Outputs/1

== system RoboBoat_SS_July3_v6/Main FSM/Obstacle Navigation1/Obstacle Navigation/Output Reassign ==
  Outputs in : Inport
  Bus Assignment : BusAssignment  AssignedSignals=Task Finished
  Bus Selector : BusSelector  OutputSignals=Task Finished
  Constant : Constant  Value=0
  Outputs : Outport
  Finished : Outport  Port=2
  wires:
  Outputs in/1 -> Bus Assignment/1, Bus Selector/1
  Bus Selector/1 -> Finished/1  "<Task Finished>"
  Bus Assignment/1 -> Outputs/1
  Constant/1 -> Bus Assignment/2

== system RoboBoat_SS_July3_v6/Main FSM/Start Speed/Gate Find and Through/Find ==
  Sensors : Inport
  Enable : EnablePort
  Bus Selector : BusSelector  OutputSignals=LIDAR.Landmarks.Distances,LIDAR.Landmarks.Angles,IMU.Position.X,IMU.Position.Y,IMU.Orientation.Yaw,LIDAR.Color data.Color,LIDAR.Color data.idx
  Data Store Read3 : DataStoreRead  DataStoreName=holdHeading
  MATLAB Function1 : MATLAB Function  TreatAsAtomicUnit=on
  Output Heirarchy : Subsystem
  RPM : Constant  Value=4000  SampleTime=-1
  Write : DataStoreWrite  DataStoreName=GateNED
  Outputs : Outport
  Finished : Outport  Port=2
  wires:
  Output Heirarchy/1(Outputs) -> Outputs/1
  RPM/1 -> Output Heirarchy/2(RPM)
  MATLAB Function1/2(Goal) -> Write/1
  MATLAB Function1/1(found) -> Finished/1
  Sensors/1 -> Output Heirarchy/1(Sensors), Bus Selector/1  "Sensors"
  Bus Selector/1 -> MATLAB Function1/1(Dist)  "<Distances>"
  Bus Selector/3 -> MATLAB Function1/3(X)  "<X>"
  Bus Selector/2 -> MATLAB Function1/2(Angles)  "<Angles>"
  Bus Selector/4 -> MATLAB Function1/4(Y)  "<Y>"
  Bus Selector/5 -> MATLAB Function1/5(Heading)  "<Yaw>"
  Data Store Read3/1 -> Output Heirarchy/3(Desired Heading)
  Bus Selector/6 -> MATLAB Function1/6(Color)  "<Color>"
  Bus Selector/7 -> MATLAB Function1/7(idx)  "<idx>"

== system RoboBoat_SS_July3_v6/Main FSM/Start Speed/Gate Find and Through/Point ==
  Sensors : Inport
  Enable : EnablePort
  Bus Selector : BusSelector  OutputSignals=IMU.Orientation.Yaw
  Data Store Read3 : DataStoreRead  DataStoreName=holdHeading
  MATLAB Function1 : MATLAB Function  TreatAsAtomicUnit=on
  Output Heirarchy : Subsystem
  RPM : Constant  Value=0  SampleTime=-1
  Outputs : Outport
  Finished : Outport  Port=2
  wires:
  Output Heirarchy/1(Outputs) -> Outputs/1
  RPM/1 -> Output Heirarchy/2(RPM)
  MATLAB Function1/1(finished) -> Finished/1
  Sensors/1 -> Bus Selector/1, Output Heirarchy/1(Sensors)
  Data Store Read3/1 -> MATLAB Function1/1(holdHeading), Output Heirarchy/3(Desired Heading)
  Bus Selector/1 -> MATLAB Function1/2(yaw)  "<Yaw>"

== system RoboBoat_SS_July3_v6/Main FSM/Start Speed/Gate Find and Through/Through ==
  Sensors : Inport
  Enable : EnablePort
  Bus Selector2 : BusSelector  OutputSignals=IMU.Position.X,IMU.Position.Y,IMU.Orientation.Yaw
  Data Store Read3 : DataStoreRead  DataStoreName=GateNED
  Demux : Demux  Outputs=2
  Model : ModelReference  ModelNameDialog=NEDnavV5.slx  SimulationMode=Normal  ModelReferenceVersion=1.2059  CopyOfModelName=NEDnavV5.slx  DefaultDataLogging=on
  Output Heirarchy : Subsystem
  Outputs : Outport
  Finished : Outport  Port=2
  wires:
  Model/1 -> Output Heirarchy/2(RPM)
  Model/2 -> Output Heirarchy/3(Desired Heading)
  Model/3 -> Finished/1
  Output Heirarchy/1(Outputs) -> Outputs/1
  Sensors/1 -> Bus Selector2/1, Output Heirarchy/1(Sensors)
  Bus Selector2/1 -> Model/1  "<X>"
  Bus Selector2/2 -> Model/2  "<Y>"
  Bus Selector2/3 -> Model/3  "<Yaw>"
  Data Store Read3/1 -> Demux/1
  Demux/1 -> Model/4
  Demux/2 -> Model/5

== system RoboBoat_SS_July3_v6/Main FSM/Start Speed/Gate Find and Through1/Find ==
  Sensors : Inport
  Enable : EnablePort
  Bus Selector : BusSelector  OutputSignals=LIDAR.Landmarks.Distances,LIDAR.Landmarks.Angles,IMU.Position.X,IMU.Position.Y,IMU.Orientation.Yaw,LIDAR.Color data.Color,LIDAR.Color data.idx
  Data Store Read3 : DataStoreRead  DataStoreName=holdHeading
  MATLAB Function1 : MATLAB Function  TreatAsAtomicUnit=on
  Output Heirarchy : Subsystem
  RPM : Constant  Value=4000  SampleTime=-1
  Write : DataStoreWrite  DataStoreName=GateNED
  Outputs : Outport
  Finished : Outport  Port=2
  wires:
  Output Heirarchy/1(Outputs) -> Outputs/1
  RPM/1 -> Output Heirarchy/2(RPM)
  MATLAB Function1/2(Goal) -> Write/1
  MATLAB Function1/1(found) -> Finished/1
  Sensors/1 -> Output Heirarchy/1(Sensors), Bus Selector/1  "Sensors"
  Bus Selector/1 -> MATLAB Function1/1(Dist)  "<Distances>"
  Bus Selector/3 -> MATLAB Function1/3(X)  "<X>"
  Bus Selector/2 -> MATLAB Function1/2(Angles)  "<Angles>"
  Bus Selector/4 -> MATLAB Function1/4(Y)  "<Y>"
  Bus Selector/5 -> MATLAB Function1/5(Heading)  "<Yaw>"
  Data Store Read3/1 -> Output Heirarchy/3(Desired Heading)
  Bus Selector/6 -> MATLAB Function1/6(Color)  "<Color>"
  Bus Selector/7 -> MATLAB Function1/7(idx)  "<idx>"

== system RoboBoat_SS_July3_v6/Main FSM/Start Speed/Gate Find and Through1/Point ==
  Sensors : Inport
  Enable : EnablePort
  Bus Selector : BusSelector  OutputSignals=IMU.Orientation.Yaw
  Data Store Read3 : DataStoreRead  DataStoreName=holdHeading
  MATLAB Function1 : MATLAB Function  TreatAsAtomicUnit=on
  Output Heirarchy : Subsystem
  RPM : Constant  Value=0  SampleTime=-1
  Outputs : Outport
  Finished : Outport  Port=2
  wires:
  Output Heirarchy/1(Outputs) -> Outputs/1
  RPM/1 -> Output Heirarchy/2(RPM)
  MATLAB Function1/1(finished) -> Finished/1
  Sensors/1 -> Bus Selector/1, Output Heirarchy/1(Sensors)
  Data Store Read3/1 -> MATLAB Function1/1(holdHeading), Output Heirarchy/3(Desired Heading)
  Bus Selector/1 -> MATLAB Function1/2(yaw)  "<Yaw>"
